simulink model "model"  (R2018b)
settings: Solver=VariableStepAuto  StartTime=0.0  StopTime=10  RelTol=1e-3
values from neighbouring files (symbols this model uses):
  Alpha = 0.007    [model_init.m]
  Beta = 0.05    [model_init.m]
  Ce = 0.132    [model_init.m]
  Cm = 30*Ce/pi    (= 1.26050714929)    [model_init.m]
  gain = 100    [model_init.m]
  Jg = GD2*30/(375*pi)    (= 0.700281749604)    [model_init.m]
  Ki = 1.875    [model_init.m]
  Kn = 12.1    [model_init.m]
  Ks = 40    [model_init.m]
  R = 0.5    [model_init.m]
  ti = 0.03    [model_init.m]
  Tl = 0.03    [model_init.m]
  tn = 0.084    [model_init.m]
  Toi = 0.002    [model_init.m]
  Ton = 0.01    [model_init.m]
libraries: powerlib x1
settings Model: Creator=12516  LastModifiedBy=12516

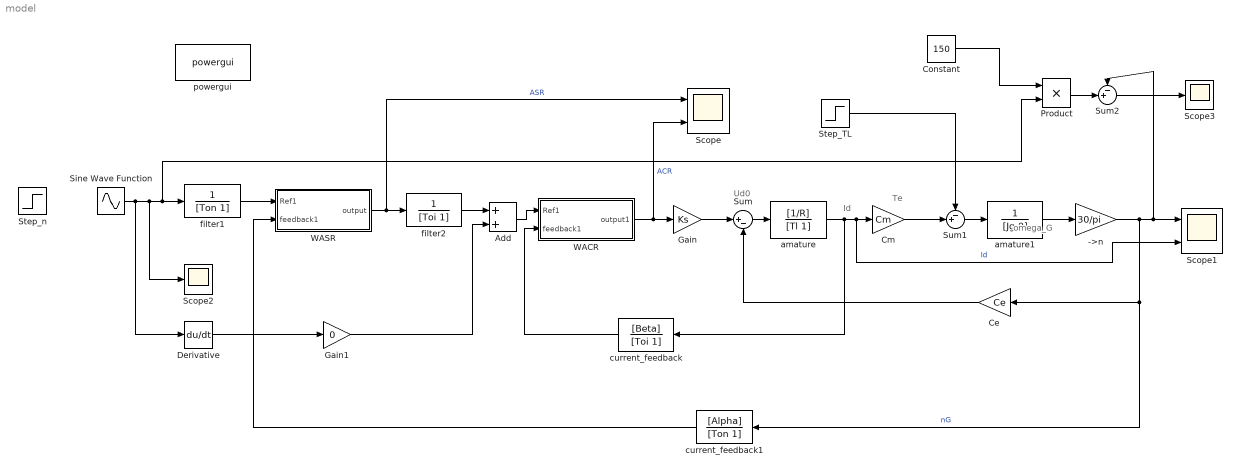
== system model ==
  note: Id
  note: Ud0
  note: Te
  note: omega_G
  ->n : Gain  Gain=30/pi
  Add : Sum
  Ce : Gain  Gain=Ce
  Cm : Gain  Gain=Cm
  Constant : Constant  Value=150
  Derivative : Derivative
  Gain : Gain  Gain=Ks
  Gain1 : Gain  Gain=0
  Product : Product
  Scope : Scope  NumInputPorts=2
  Scope1 : Scope  NumInputPorts=2
  Scope2 : Scope
  Scope3 : Scope
  Sine Wave Function : Sin  Frequency=5  SampleTime=0
  Step_TL : Step  Time=7  After=100  SampleTime=0
  Step_n : Step  Time=2  After=10.22  SampleTime=0
  Sum : Sum  Inputs=|+-
  Sum1 : Sum  Inputs=-+|
  Sum2 : Sum  Inputs=-+|
  WACR : Subsystem
  WASR : Subsystem
  amature : TransferFcn  Numerator=[1/R]  Denominator=[Tl 1]
  amature1 : TransferFcn  Denominator=[Jg 0]
  current_feedback : TransferFcn  Numerator=[Beta]  Denominator=[Toi 1]
  current_feedback1 : TransferFcn  Numerator=[Alpha]  Denominator=[Ton 1]
  filter1 : TransferFcn  Denominator=[Ton 1]
  filter2 : TransferFcn  Denominator=[Toi 1]
  powergui : powerlib/powergui  Priority=1  SimulationMode=Continuous  SampleTime=50e-6  frequency=60  Iterations=50  frequencyindice=60  Pbase=100e6  ErrMax=1e-4  UnitsV=kV  UnitsW=MW  buscounter=0  FunctionMessages=off  echomessages=off  EnableUseOfTLC=off  CurrentSourceSwitches=off  DisableSnubberDevices=off  DisableRonSwitches=off  DisableVfSwitches=off  DisplayEquations=off  SolverType=Tustin/Backward Euler (TBE)  Interpol=off  ExternalGateDelay=off  methode=off  Ts=100  x0status=blocks  SPID=on  SwTol=0  HookPort=off  RestoreLinks=warning  ResistiveCurrentMeasurement=off  Frange=[0:2:500]  Ylog=off  Xlog=on  ShowGrid=off  save=off  variable=ZData  structure=0  ZoomFFT=off  StartTime=0.0  cycles=1  DisplayStyle=1  fundamental=60  FreqAxis=off  MaxFrequency=1000  frequencyindicesteady=1  RmsSteady=1  display=off
  wires:
  WASR/1(output) -> filter2/1, Scope/1  "ASR"
  WACR/1(output1) -> Scope/2, Gain/1  "ACR"
  Step_TL/1 -> Sum1/1
  current_feedback/1 -> WACR/2(feedback1)
  filter1/1 -> WASR/1(Ref1)
  amature1/1 -> ->n/1
  current_feedback1/1 -> WASR/2(feedback1)
  Cm/1 -> Sum1/2
  Ce/1 -> Sum/2
  amature/1 -> Scope1/2, Cm/1, current_feedback/1  "Id"
  ->n/1 -> Sum2/1, Scope1/1, Ce/1, current_feedback1/1  "nG"
  Sum1/1 -> amature1/1
  Sum/1 -> amature/1
  Gain/1 -> Sum/1
  Sine Wave Function/1 -> Derivative/1, Scope2/1, Product/2, filter1/1
  Sum2/1 -> Scope3/1
  Product/1 -> Sum2/2
  Constant/1 -> Product/1
  filter2/1 -> Add/1
  Add/1 -> WACR/1(Ref1)
  Derivative/1 -> Gain1/1
  Gain1/1 -> Add/2

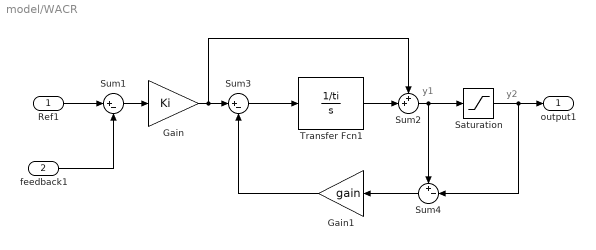
== system model/WACR ==
  note: y2
  note: y1
  Ref1 : Inport
  feedback1 : Inport  Port=2
  Gain : Gain  Gain=Ki
  Gain1 : Gain  Gain=gain
  Saturation : Saturate  UpperLimit=10  LowerLimit=-10
  Sum1 : Sum  Inputs=|+-
  Sum2 : Sum  Inputs=++|
  Sum3 : Sum  Inputs=|+-
  Sum4 : Sum  Inputs=+-|
  Transfer Fcn1 : TransferFcn  Numerator=1/ti  Denominator=[1 0]
  output1 : Outport
  wires:
  Ref1/1 -> Sum1/1
  Gain/1 -> Sum2/1, Sum3/1
  Sum3/1 -> Transfer Fcn1/1
  Transfer Fcn1/1 -> Sum2/2
  Sum2/1 -> Saturation/1, Sum4/1
  Saturation/1 -> output1/1, Sum4/2
  Sum4/1 -> Gain1/1
  Gain1/1 -> Sum3/2
  Sum1/1 -> Gain/1
  feedback1/1 -> Sum1/2

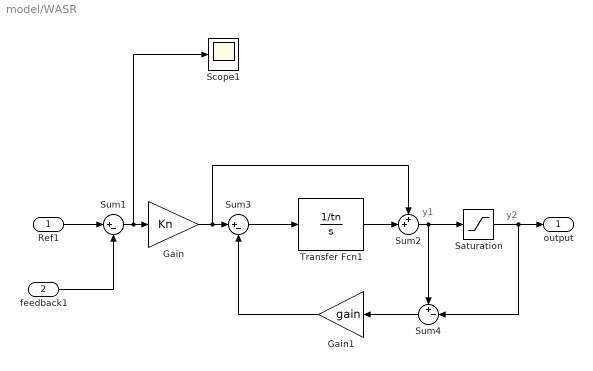
== system model/WASR ==
  note: y2
  note: y1
  Ref1 : Inport
  feedback1 : Inport  Port=2
  Gain : Gain  Gain=Kn
  Gain1 : Gain  Gain=gain
  Saturation : Saturate  UpperLimit=10  LowerLimit=-10
  Scope1 : Scope
  Sum1 : Sum  Inputs=|+-
  Sum2 : Sum  Inputs=++|
  Sum3 : Sum  Inputs=|+-
  Sum4 : Sum  Inputs=+-|
  Transfer Fcn1 : TransferFcn  Numerator=1/tn  Denominator=[1 0]
  output : Outport
  wires:
  Ref1/1 -> Sum1/1
  Sum3/1 -> Transfer Fcn1/1
  Transfer Fcn1/1 -> Sum2/2
  Sum2/1 -> Saturation/1, Sum4/1
  Saturation/1 -> output/1, Sum4/2
  Sum4/1 -> Gain1/1
  Gain1/1 -> Sum3/2
  Sum1/1 -> Gain/1, Scope1/1
  feedback1/1 -> Sum1/2
  Gain/1 -> Sum2/1, Sum3/1
